simulink model "cruise_sys"  (R2021a)
settings: Solver=FixedStepDiscrete  StartTime=0.0  StopTime=inf  FixedStep=0.01  MaxStep=1e-3  RelTol=1e-3
settings Model: EnablePacing=on  Creator=AHMED  LastModifiedBy=AHMED

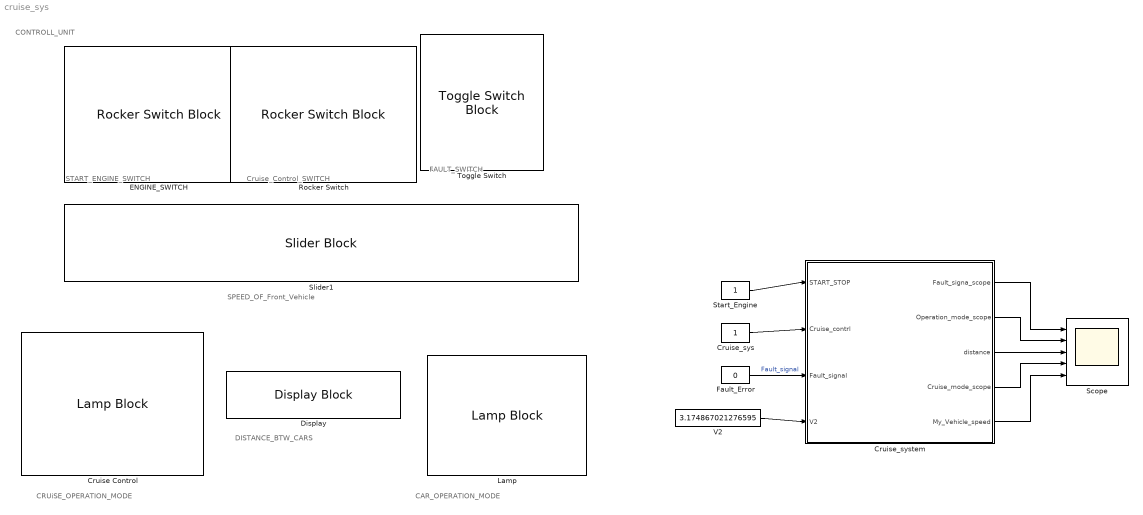
== system cruise_sys ==
  note: START_ENGINE_SWITCH
  note: CONTROLL_UNIT
  note: Cruise_Control_SWITCH
  note: FAULT_SWITCH
  note: SPEED_OF_Front_Vehicle
  note: CRUiSE_OPERATION_MODE
  note: CAR_OPERATION_MODE
  note: DISTANCE_BTW_CARS
  Cruise Control : LampBlock  LabelPosition=Bottom  Icon=CruiseControl
  Cruise_sys : Constant
  Cruise_system : Subsystem
  Display : DisplayBlock  LabelPosition=Hide  Format=short  Transparency=1
  ENGINE_SWITCH : RockerSwitchBlock
      settings: Values={{'Off', 'On'}, [0 1]}
  Fault_Error : Constant  Value=0
  Lamp : LampBlock
  Rocker Switch : RockerSwitchBlock
      settings: Values={{'Off', 'On'}, [0 1]}
  Scope : Scope  NumInputPorts=5
  Slider1 : SliderBlock  ScaleMax=20
  Start_Engine : Constant
  Toggle Switch : ToggleSwitchBlock
      settings: Values={{'Off', 'On'}, [0 1]}
  V2 : Constant  Value=3.174867021276595
  wires:
  Start_Engine/1 -> Cruise_system/1(START_STOP)
  Cruise_sys/1 -> Cruise_system/2(Cruise_contrl)
  Fault_Error/1 -> Cruise_system/3(Fault_signal)  "Fault_signal"
  Cruise_system/1(Fault_signa_scope) -> Scope/1
  Cruise_system/2(Operation_mode_scope) -> Scope/2
  Cruise_system/3(distance) -> Scope/3
  Cruise_system/4(Cruise_mode_scope) -> Scope/4
  V2/1 -> Cruise_system/4(V2)
  Cruise_system/5(My_Vehicle_speed) -> Scope/5

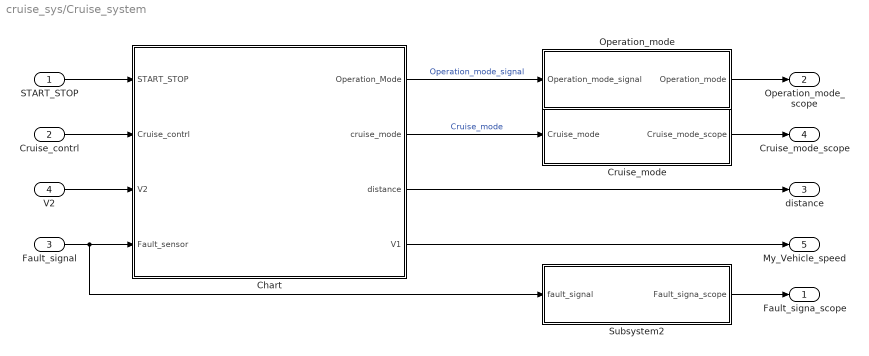
== system cruise_sys/Cruise_system ==
  START_STOP : Inport
  Cruise_contrl : Inport  Port=2
  Fault_signal : Inport  Port=3
  V2 : Inport  Port=4
  Chart : Stateflow chart  TreatAsAtomicUnit=on
  Cruise_mode : Subsystem
  Operation_mode : Subsystem
  Subsystem2 : Subsystem
  Fault_signa_scope : Outport
  Operation_mode_scope : Outport  Port=2
  distance : Outport  Port=3
  Cruise_mode_scope : Outport  Port=4
  My_Vehicle_speed : Outport  Port=5
  wires:
  Cruise_contrl/1 -> Chart/2(Cruise_contrl)
  Chart/3(distance) -> distance/1
  Fault_signal/1 -> Subsystem2/1(fault_signal), Chart/4(Fault_sensor)
  START_STOP/1 -> Chart/1(START_STOP)
  Chart/1(Operation_Mode) -> Operation_mode/1(Operation_mode_signal)  "Operation_mode_signal"
  Operation_mode/1(Operation_mode) -> Operation_mode_scope/1
  Chart/2(cruise_mode) -> Cruise_mode/1(Cruise_mode)  "Cruise_mode"
  Cruise_mode/1(Cruise_mode_scope) -> Cruise_mode_scope/1
  Subsystem2/1(Fault_signa_scope) -> Fault_signa_scope/1
  V2/1 -> Chart/3(V2)
  Chart/4(V1) -> My_Vehicle_speed/1

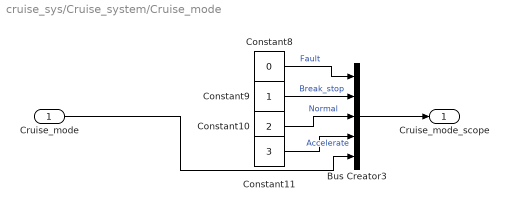
== system cruise_sys/Cruise_system/Cruise_mode ==
  Cruise_mode : Inport
  Bus Creator3 : BusCreator  Inputs=5
  Constant10 : Constant  Value=2
  Constant11 : Constant  Value=3
  Constant8 : Constant  Value=0
  Constant9 : Constant
  Cruise_mode_scope : Outport
  wires:
  Bus Creator3/1 -> Cruise_mode_scope/1
  Cruise_mode/1 -> Bus Creator3/5
  Constant10/1 -> Bus Creator3/3  "Normal"
  Constant8/1 -> Bus Creator3/1  "Fault"
  Constant9/1 -> Bus Creator3/2  "Break_stop"
  Constant11/1 -> Bus Creator3/4  "Accelerate"

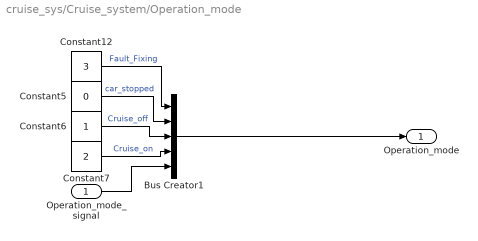
== system cruise_sys/Cruise_system/Operation_mode ==
  Operation_mode_signal : Inport
  Bus Creator1 : BusCreator  Inputs=5
  Constant12 : Constant  Value=3
  Constant5 : Constant  Value=0
  Constant6 : Constant
  Constant7 : Constant  Value=2
  Operation_mode : Outport
  wires:
  Constant6/1 -> Bus Creator1/3  "Cruise_off"
  Operation_mode_signal/1 -> Bus Creator1/5
  Bus Creator1/1 -> Operation_mode/1
  Constant5/1 -> Bus Creator1/2  "car_stopped"
  Constant12/1 -> Bus Creator1/1  "Fault_Fixing"
  Constant7/1 -> Bus Creator1/4  "Cruise_on"

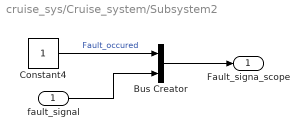
== system cruise_sys/Cruise_system/Subsystem2 ==
  fault_signal : Inport
  Bus Creator : BusCreator  Inputs=2
  Constant4 : Constant
  Fault_signa_scope : Outport
  wires:
  fault_signal/1 -> Bus Creator/2
  Constant4/1 -> Bus Creator/1  "Fault_occured"
  Bus Creator/1 -> Fault_signa_scope/1

== stateflow chart cruise_sys/Cruise_system/Chart ==
  state Car_Start
    state Crusie_Control_on
      state Normal_operating
        en:Operation_Mode=App_modes.cruise_on;
        state Distance_Measuring
          en:
          distance=default_distance;
          du:
          distance=default_distance;
        state Accelerate
          en:
          distance=distance-(V1-V2);
          default_distance=distance;
          cruise_mode=App_modes.Accelerate;
        state No_thing
          en:
          cruise_mode=App_modes.No_thing;
          distance=distance-(V1-V2);
          default_distance=distance;
        state Stop
          en:
          cruise_mode=App_modes.break_stop;
        (default) -> Distance_Measuring
        Distance_Measuring -> Accelerate [order 2] : [(distance >10)&&(V1<=V2)]{V1++;}
        Distance_Measuring -> Accelerate [order 1] : [(distance >10)&&(V1>V2)]
        Accelerate -> Distance_Measuring [order 2] : after(100,tick)
        Accelerate -> Distance_Measuring [order 1] : after(100,tick)[(distance <=10)]{V1=V2;}
        No_thing -> Distance_Measuring : after(100,tick)
        Distance_Measuring -> No_thing [order 3] : [(distance <=10)&&(distance >=5)]
        Distance_Measuring -> Stop [order 4] : [distance <5]
        Stop -> Distance_Measuring : after(100,tick)
      state Fault
        en:
        fault_counter=0;
        du:
        Operation_Mode=App_modes.cruise_fault;
        cruise_mode=App_modes.cruise_fault2;
        fault_counter++;
      (default) -> Normal_operating
      Fault -> Normal_operating [order 1] : [(Fault_sensor==0)&&(fault_counter<500)]
      Normal_operating -> Fault : [Fault_sensor==1]
    state Crusie_Control_off
      during:
      Operation_Mode=App_modes.cruise_off;
    state Crusie_Control_off1
      during:
      Operation_Mode=App_modes.cruise_off2;
    (default) -> Crusie_Control_on
    Crusie_Control_on -> Crusie_Control_off : [Cruise_contrl==0]
    Crusie_Control_off -> Crusie_Control_on : [Cruise_contrl==1]
    Fault -> Crusie_Control_off1 [order 2] : [(Fault_sensor==1)&&(fault_counter >500)]
  state Car_Stop
    du:
    Operation_Mode=App_modes.Car_stoped;
  (default) -> Car_Start
  Car_Start -> Car_Stop : [START_STOP==0]
  Car_Stop -> Car_Start : [START_STOP==1]
  data: START_STOP input; Operation_Mode output double; Cruise_contrl input; fault_counter local double; cruise_mode output double; distance output double; V2 input double =11; Fault_sensor input; default_distance local double =15; V1 output double =10
